simulink model "modules_intentions"  (R2017a)
settings: Solver=ode4  StartTime=0.0  StopTime=time_stop  FixedStep=time_step  RelTol=1e-3
undefined symbols (not defined in the file or in its folder): beta, Delta_guidance, Delta_matrix, eta_initial, initial_desired_psi_vector, initial_desired_u_vector, initial_next_waypoint_indexes, initial_obstacle_ship_states, initial_obstacle_ship_states_dot, initial_reference_psi_vector, initial_reference_u_vector, initial_SBMPC_desired_psi_vector, initial_SBMPC_desired_u_vector, initial_SBMPC_next_waypoint_indexes, initial_SBMPC_obstacle_ship_states, initial_SBMPC_obstacle_ship_states_dot, initial_SBMPC_reference_psi_vector, initial_SBMPC_reference_u_vector, initial_SBMPC_x_d_psi_matrix, initial_SBMPC_x_d_u_matrix, initial_state, initial_x_d_psi_matrix, initial_x_d_u_matrix, K_sway, K_yaw, Kp_feedback_linearization, kp_heading, Nmax, nu_initial, num_obs_ship_waypoints, num_prediction_time_steps, number_of_control_behaviors, number_of_obstacle_ships, number_of_SBMPC_obstacle_ships, obs_speed_between_waypoints, obstacle_waypoint_matrix, Omega_matrix, own_ship_reference_psi_init, own_ship_reference_speed, psi, Psi_init, radius_of_acceptance, SBMPC_obs_speed_between_waypoints, SBMPC_obstacle_waypoint_matrix, seconds_between_prediction, state_vector_init, T, T_k_surge, T_k_sway, T_k_yaw, T_s, T_waypoints, time_step, tsamp, U, U_init, V_init, waypoints_obstacle_ships, waypoints_own_ship, Xmax ... (+1)
(part 4 of 6)

== matlab function modules_intentions/SBMPC obstacle ships/SBMPC using intentions /Calculate control behaviors/Compute hazard ==
  settings: updateMethod=DISCRETE  sampleTime=time_step
  data: obstacle_ships_u_input input size=[1 + number_of_obstacle_ships, num_prediction_time_steps]; obstacle_ships_v_input input size=[1 + number_of_obstacle_ships, num_prediction_time_steps]; obstacle_ships_psi_input input size=[1 + number_of_obstacle_ships, num_prediction_time_steps]; t_0 input; SBMPC_obstacles_own_ship_x_predicted input size=[number_of_SBMPC_obstacle_ships, num_prediction_time_steps, number_of_control_behaviors]; SBMPC_obstacles_own_ship_y_predicted input size=[number_of_SBMPC_obstacle_ships, num_prediction_time_steps, number_of_control_behaviors]; SBMPC_obstacles_own_ship_u_predicted input size=[number_of_SBMPC_obstacle_ships, num_prediction_time_steps, number_of_control_behaviors]; SBMPC_obstacles_own_ship_v_predicted input size=[number_of_SBMPC_obstacle_ships, num_prediction_time_steps, number_of_control_behaviors]; SBMPC_obstacles_own_ship_heading_predicted input size=[number_of_SBMPC_obstacle_ships, num_prediction_time_steps, number_of_control_behaviors]; CLOSE output size=[number_of_SBMPC_obstacle_ships, number_of_control_behaviors, total_number_of_obstacle_ships, num_prediction_time_steps]; d_0 output size=[number_of_SBMPC_obstacle_ships, number_of_control_behaviors, total_number_of_obstacle_ships, num_prediction_time_steps]; obstacle_ships_x_predicted_input input size=[1 + number_of_obstacle_ships, num_prediction_time_steps]; obstacle_ships_y_predicted_input input size=[1 + number_of_obstacle_ships, num_prediction_time_steps]; OVERTAKEN output size=[number_of_SBMPC_obstacle_ships, number_of_control_behaviors, total_number_of_obstacle_ships, num_prediction_time_steps]; STARBOARD output size=[number_of_SBMPC_obstacle_ships, number_of_control_behaviors, total_number_of_obstacle_ships, num_prediction_time_steps]; chosen_HEAD_ON_out output; CROSSED output size=[number_of_SBMPC_obstacle_ships, number_of_control_behaviors, total_number_of_obstacle_ships, num_prediction_time_steps]; mu output size=[number_of_SBMPC_obstacle_ships, number_of_control_behaviors, total_number_of_obstacle_ships, num_prediction_time_steps]; num_prediction_time_steps parameter; heading_angle_offset_commands parameter; propulsion_commands parameter; total_number_of_obstacle_ships parameter; seconds_between_prediction parameter; d_cl parameter; phi_head_on parameter; phi_crossed parameter; phi_overtaken parameter; phi_ahead parameter; K_coll parameter; C output size=[number_of_SBMPC_obstacle_ships, number_of_control_behaviors, total_number_of_obstacle_ships, num_prediction_time_steps]; R output size=[number_of_SBMPC_obstacle_ships, number_of_control_behaviors, total_number_of_obstacle_ships, num_prediction_time_steps]; q parameter; p parameter; d_safe parameter; k_boundary parameter; k_circle parameter; k_Pr parameter; k_psi_port parameter; k_psi_starboard parameter; Delta_Pr parameter; vessel_length parameter; circle_obstacle_parameters parameter; boundary_obstacles_parameters parameter; k_Delta_psi_port parameter; k_Delta_psi_starboard parameter; kappa parameter; f output size=[number_of_SBMPC_obstacle_ships,number_of_control_behaviors]; g output size=[number_of_SBMPC_obstacle_ships,number_of_control_behaviors]; hazard output size=[number_of_SBMPC_obstacle_ships,number_of_control_behaviors]; rad2deg parameter; num_boundary_obstacles parameter; num_circle_obstacles parameter; chosen_C_out output; chosen_P_out output; chosen_FC_out output; chosen_R_out output; chosen_scaled_mu_out output; T_s parameter; chosen_Pr_out output; chosen_psi_ca_out output; C_worst output; R_worst output; scaled_mu_worst output; Pr_worst output; psi_ca_worst output; f_worst_out output; g_worst_out output; smallest_hazard_out output; largest_hazard_out output; f_out output; g_out output; r parameter; L_C input; circle_safety_margin parameter; p_boundary parameter; p_circle parameter; q_circle parameter; q_boundary parameter; boundary_margin parameter; k_role parameter; L_role parameter; ROLE_relative_to_SBMPC_obs_module parameter; L_FC parameter; k_FC parameter; number_of_control_behaviors parameter; HEAD_ON_relative_to_SBMPC_obs_module parameter; chosen_scenario_index_out output; number_of_SBMPC_obstacle_ships parameter; chosen_scenario_index_out_init parameter; data_out_init parameter; number_of_obstacle_ships parameter; HEAD_ON_SBMPC_relative_to_SBMPC_obs parameter; ROLE_SBMPC_relative_to_SBMPC_obs parameter
function [CLOSE, d_0, OVERTAKEN, STARBOARD, chosen_HEAD_ON_out, CROSSED,mu, C, R, f, g, hazard, chosen_C_out, chosen_P_out, chosen_FC_out, chosen_R_out, chosen_scaled_mu_out, chosen_Pr_out, chosen_psi_ca_out, C_worst, R_worst, scaled_mu_worst, Pr_worst, psi_ca_worst, f_worst_out, g_worst_out, smallest_hazard_out, largest_hazard_out, f_out, g_out, chosen_scenario_index_out]                         = computeTotalHazard(obstacle_ships_u_input, obstacle_ships_v_input, obstacle_ships_psi_input, t_0,SBMPC_obstacles_own_ship_x_predicted, SBMPC_obstacles_own_ship_y_predicted,SBMPC_obstacles_own_ship_u_predicted,SBMPC_obstacles_own_ship_v_predicted, SBMPC_obstacles_own_ship_heading_predicted, obstacle_ships_x_predicted_input, obstacle_ships_y_predicted_input, num_prediction_time_steps, heading_angle_offset_commands, propulsion_commands, total_number_of_obstacle_ships, seconds_between_prediction, d_cl,phi_head_on, phi_crossed, phi_overtaken,phi_ahead,K_coll, q, p, d_safe,k_boundary, k_circle, k_Pr, k_psi_port, k_psi_starboard, Delta_Pr, vessel_length, circle_obstacle_parameters, boundary_obstacles_parameters, k_Delta_psi_port, k_Delta_psi_starboard,kappa, rad2deg, num_boundary_obstacles, num_circle_obstacles, T_s, r, L_C,  circle_safety_margin, p_boundary, p_circle, q_circle, q_boundary, boundary_margin, k_role, L_role, ROLE_relative_to_SBMPC_obs_module, L_FC, k_FC, number_of_control_behaviors, HEAD_ON_relative_to_SBMPC_obs_module, number_of_SBMPC_obstacle_ships, chosen_scenario_index_out_init, data_out_init, number_of_obstacle_ships, HEAD_ON_SBMPC_relative_to_SBMPC_obs, ROLE_SBMPC_relative_to_SBMPC_obs)     
    
    persistent chosen_C;
    persistent chosen_scenario_index;
    persistent chosen_R;
    persistent chosen_scaled_mu;
    persistent chosen_P_role;
    persistent chosen_FC;
    persistent chosen_HEAD_ON;
    persistent chosen_Pr;
    persistent chosen_psi_ca;
    persistent chosen_Pr_worst;
    persistent chosen_psi_ca_worst;
    persistent f_worst;
    persistent g_worst;
    persistent f_chosen;
    persistent g_chosen;
    persistent smallest_hazard;
    persistent largest_hazard;
    persistent scenario_index_with_min_hazard;
    persistent scenario_index_with_max_hazard;
    
    if (isempty(chosen_C))
        chosen_C              = zeros(number_of_SBMPC_obstacle_ships,number_of_control_behaviors);%chosen_C_init;
        chosen_scenario_index = ones(1,number_of_SBMPC_obstacle_ships)*7;
        chosen_R              = zeros(number_of_SBMPC_obstacle_ships,number_of_control_behaviors);%chosen_R_init;
        chosen_scaled_mu      = zeros(number_of_SBMPC_obstacle_ships,number_of_control_behaviors);%chosen_scaled_mu_init; 
        chosen_P_role         = zeros(number_of_SBMPC_obstacle_ships,number_of_control_behaviors);%chosen_P_role_init;
        chosen_FC             = zeros(number_of_SBMPC_obstacle_ships,number_of_control_behaviors);
        chosen_HEAD_ON        = zeros(number_of_SBMPC_obstacle_ships,number_of_control_behaviors);
        chosen_Pr             = ones(1, number_of_SBMPC_obstacle_ships);
        chosen_psi_ca         = data_out_init;
        chosen_Pr_worst       = data_out_init;
        chosen_psi_ca_worst   = data_out_init;
        f_worst               = data_out_init;
        g_worst               = data_out_init;
        f_chosen              = data_out_init;
        g_chosen              = data_out_init;
        smallest_hazard       = data_out_init;
        largest_hazard        = data_out_init;
        scenario_index_with_min_hazard = ones(1, number_of_SBMPC_obstacle_ships)*(-1);
        scenario_index_with_max_hazard = ones(1, number_of_SBMPC_obstacle_ships)*(-1);
        
    end
    
    chosen_scenario_index_out = chosen_scenario_index_out_init;

    CLOSE     = zeros(number_of_SBMPC_obstacle_ships, number_of_control_behaviors, total_number_of_obstacle_ships, num_prediction_time_steps);
    OVERTAKEN = zeros(number_of_SBMPC_obstacle_ships, number_of_control_behaviors, total_number_of_obstacle_ships, num_prediction_time_steps);
    STARBOARD = zeros(number_of_SBMPC_obstacle_ships, number_of_control_behaviors, total_number_of_obstacle_ships, num_prediction_time_steps);
    HEAD_ON   = zeros(number_of_SBMPC_obstacle_ships, number_of_control_behaviors, total_number_of_obstacle_ships, num_prediction_time_steps);
    CROSSED   = zeros(number_of_SBMPC_obstacle_ships, number_of_control_behaviors, total_number_of_obstacle_ships, num_prediction_time_steps);
    mu        = zeros(number_of_SBMPC_obstacle_ships, number_of_control_behaviors, total_number_of_obstacle_ships, num_prediction_time_steps);
    scaled_mu = zeros(number_of_SBMPC_obstacle_ships, number_of_control_behaviors, total_number_of_obstacle_ships, num_prediction_time_steps);
    d_0       = zeros(number_of_SBMPC_obstacle_ships, number_of_control_behaviors, total_number_of_obstacle_ships, num_prediction_time_steps);
    f         = zeros(number_of_SBMPC_obstacle_ships,number_of_control_behaviors);
    g         = zeros(number_of_SBMPC_obstacle_ships,number_of_control_behaviors);
    chosen_HEAD_ON_out   = data_out_init;
    chosen_C_out         = data_out_init;
    chosen_P_out         = data_out_init;
    chosen_FC_out        = data_out_init;
    chosen_R_out         = data_out_init;
    chosen_scaled_mu_out =data_out_init;
    chosen_Pr_out        = data_out_init;
    chosen_psi_ca_out    = data_out_init;
    C_worst              = data_out_init;
    P_worst              = data_out_init;
    R_worst              = data_out_init;
    scaled_mu_worst      = data_out_init;
    Pr_worst             = data_out_init;
    psi_ca_worst         =data_out_init;
    f_worst_out          = data_out_init;
    g_worst_out          = data_out_init;
    smallest_hazard_out  = data_out_init;
    largest_hazard_out   = data_out_init;
    f_out                = data_out_init;
    g_out                = data_out_init;
    %R_vector_out         = zeros(number_of_control_behaviors, total_number_of_obstacle_ships, num_prediction_time_steps, number_of_SBMPC_obstacle_ships);
    %chosen_scenario_index_out  = zeros(1, number_of_SBMPC_obstacle_ships);
    %own_ship_u_predicted       = zeros(number_of_SBMPC_obstacle_ships, num_prediction_time_steps, number_of_control_behaviors);
    %own_ship_v_predicted       = zeros(num_prediction_time_steps, number_of_control_behaviors, number_of_SBMPC_obstacle_ships);
    %own_ship_heading_predicted = zeros(num_prediction_time_steps, number_of_control_behaviors, number_of_SBMPC_obstacle_ships);
    %own_ship_x_predicted       = zeros(num_prediction_time_steps, number_of_control_behaviors, number_of_SBMPC_obstacle_ships);
    %own_ship_y_predicted       = zeros(num_prediction_time_steps, number_of_control_behaviors, number_of_SBMPC_obstacle_ships);  
    
    obstacle_ships_u           = zeros(num_prediction_time_steps, total_number_of_obstacle_ships );
    obstacle_ships_v           = zeros(num_prediction_time_steps, total_number_of_obstacle_ships );
    obstacle_ships_psi         = zeros(num_prediction_time_steps, total_number_of_obstacle_ships );
    obstacle_ships_x_predicted = zeros(num_prediction_time_steps, total_number_of_obstacle_ships);
    obstacle_ships_y_predicted = zeros(num_prediction_time_steps, total_number_of_obstacle_ships);
    
    if (num_circle_obstacles > 0)
        g_circle_init  = zeros(number_of_control_behaviors, num_circle_obstacles, num_prediction_time_steps);
    else
        g_circle_init = 0;
    end    
    if (num_boundary_obstacles > 0)
        g_boundary_init = zeros(number_of_control_behaviors, num_boundary_obstacles, num_prediction_time_steps);
    else
        g_boundary_init = 0;
    end 
    g_circle  = g_circle_init;       %3D matrix. 1. dim = scneario, 2. dim = circle obstacle index, 3. dim = prediction horizon time step.
    g_boundary = g_boundary_init;    %3D matrix. 1. dim = scneario, 2. dim = circle obstacle index, 3. dim = prediction horizon time step.
    C = zeros(number_of_SBMPC_obstacle_ships, number_of_control_behaviors, total_number_of_obstacle_ships, num_prediction_time_steps);%C_init; %cost of collision. 3D matrix, 1. dim: scenario, 2. dim: obstacle, 3. dim: prediction horizon time step.
    R = zeros(number_of_SBMPC_obstacle_ships, number_of_control_behaviors, total_number_of_obstacle_ships, num_prediction_time_steps);%R_init; %Risk of collision. 3D matrix, 1. dim: scenario, 2. dim: obstacle, 3. dim: prediction horizon time step.
    hazard = zeros(number_of_SBMPC_obstacle_ships,number_of_control_behaviors); %hazard_init;
    P_role = zeros(number_of_SBMPC_obstacle_ships, number_of_control_behaviors, total_number_of_obstacle_ships, num_prediction_time_steps);%P_role_init;
    FC     = zeros(number_of_SBMPC_obstacle_ships, number_of_control_behaviors, total_number_of_obstacle_ships, num_prediction_time_steps);%FC_init;   
    
    Pr_last = chosen_Pr;     %the Pr corresponding to the previously calculated lowest hazard.
    psi_ca_last = chosen_psi_ca;    
    if (t_0 == 0)
        Pr_last = ones(1, number_of_SBMPC_obstacle_ships);
        psi_ca_last = zeros(1, number_of_SBMPC_obstacle_ships);
    end
    prev_chosen_scenario_index = chosen_scenario_index;
    
    
    ROLE_total    = zeros(number_of_SBMPC_obstacle_ships, total_number_of_obstacle_ships);
    HEAD_ON_total = zeros(number_of_SBMPC_obstacle_ships, total_number_of_obstacle_ships);
    
    if (mod(t_0, seconds_between_prediction) == 0) %only compute every 10th second.
        
        for SBMPC_own_ship_index = 1:number_of_SBMPC_obstacle_ships
           %add SBMPC obstacle ships' data to obsatcle ship data for all sbmpc obstacle vessels except for SBMPC_own_ship_index.
           %obs data: x_predicted, y_predicted, psi, u, v, 
           %obs ship data from function "combine normal obs and own-ship obs ship data" contains own-ship module's vessel data as first element, then normal obs data, and sbmpc obstacle's data can be added at the end. 
           
           index_list = [1:number_of_SBMPC_obstacle_ships];
           SBMPC_obstacle_indexes = index_list(:,[1:(SBMPC_own_ship_index-1),(SBMPC_own_ship_index+1):end]);  %list of index values of all SBMPC obstacles EXCEPT for the SBMPC obstacle chosen to be the own-ship. 
           
           predicted_data_size = size(obstacle_ships_x_predicted_input);
           SBMPC_obs_starting_index = predicted_data_size(1);       % = 1 (own ship) + number of normal obs ships.    
           
           obstacle_ships_u(:,1:SBMPC_obs_starting_index) = obstacle_ships_u_input';
           obstacle_ships_v(:,1:SBMPC_obs_starting_index) = obstacle_ships_v_input';
           obstacle_ships_psi(:,1:SBMPC_obs_starting_index) =obstacle_ships_psi_input';
           obstacle_ships_x_predicted(:,1:SBMPC_obs_starting_index) = obstacle_ships_x_predicted_input';
           obstacle_ships_y_predicted(:,1:SBMPC_obs_starting_index) = obstacle_ships_y_predicted_input';
           
           ROLE_total(SBMPC_own_ship_index, 1:(1+number_of_obstacle_ships))    = ROLE_relative_to_SBMPC_obs_module(:,SBMPC_own_ship_index)';
           HEAD_ON_total(SBMPC_own_ship_index, 1:(1+number_of_obstacle_ships)) = HEAD_ON_relative_to_SBMPC_obs_module(:,SBMPC_own_ship_index)';
          
           if (number_of_SBMPC_obstacle_ships > 1)
               counter = 0;
               for index = 1:length(SBMPC_obstacle_indexes)
                   counter = counter + 1;
                   i = SBMPC_obstacle_indexes(index);
                   obstacle_ships_u(:,SBMPC_obs_starting_index + counter)   = SBMPC_obstacles_own_ship_u_predicted(i,:,prev_chosen_scenario_index(i));
                   obstacle_ships_v(:,SBMPC_obs_starting_index + counter)   = SBMPC_obstacles_own_ship_v_predicted(i,:,prev_chosen_scenario_index(i));
                   obstacle_ships_psi(:,SBMPC_obs_starting_index + counter) = SBMPC_obstacles_own_ship_heading_predicted(i,:,prev_chosen_scenario_index(i));
                   obstacle_ships_x_predicted(:, SBMPC_obs_starting_index + counter) =  SBMPC_obstacles_own_ship_x_predicted(i,:,prev_chosen_scenario_index(i)); %one row for each prediction time step and one column for each ship
                   obstacle_ships_y_predicted(:, SBMPC_obs_starting_index + counter) =  SBMPC_obstacles_own_ship_y_predicted(i,:,prev_chosen_scenario_index(i));   
                   ROLE_total(SBMPC_own_ship_index, 1 + number_of_obstacle_ships + counter)    = ROLE_SBMPC_relative_to_SBMPC_obs(i , SBMPC_own_ship_index);   
                   HEAD_ON_total(SBMPC_own_ship_index, 1 + number_of_obstacle_ships + counter) = HEAD_ON_SBMPC_relative_to_SBMPC_obs(i , SBMPC_own_ship_index);   
               end % end for   
           end
           
           min_ROLE_values = min(ROLE_total(SBMPC_own_ship_index,:));
           %assert (min_ROLE_values(1) >= 0);
           
           own_ship_u_predicted = reshape( SBMPC_obstacles_own_ship_u_predicted(SBMPC_own_ship_index,:,:) , [num_prediction_time_steps, number_of_control_behaviors]);
           own_ship_v_predicted = reshape( SBMPC_obstacles_own_ship_v_predicted(SBMPC_own_ship_index,:,:) , [num_prediction_time_steps, number_of_control_behaviors]);
           own_ship_heading_predicted = reshape( SBMPC_obstacles_own_ship_heading_predicted(SBMPC_own_ship_index,:,:) , [num_prediction_time_steps, number_of_control_behaviors]);
           own_ship_x_predicted = reshape( SBMPC_obstacles_own_ship_x_predicted(SBMPC_own_ship_index,:,:) , [num_prediction_time_steps, number_of_control_behaviors]);
           own_ship_y_predicted = reshape( SBMPC_obstacles_own_ship_y_predicted(SBMPC_own_ship_index,:,:) , [num_prediction_time_steps, number_of_control_behaviors]);
                   
           
           scenario_index = 0;
           for Pr = propulsion_commands
               for psi_ca = heading_angle_offset_commands 
                   scenario_index = scenario_index + 1;                      
                   prediction_time = 0;
                   for t=1:num_prediction_time_steps   
                        prediction_time = t_0 + t*T_s;  
                        %Penalty for static obstacles   
                        if (num_circle_obstacles > 0)
                            circle_obs_counter = 0;
                            for circle_obstacle = circle_obstacle_parameters.'         %in each iteration, circle_obstacle is column vector with [radius; center_x; center_y]
                                circle_obs_counter = circle_obs_counter + 1;
                                radius    = circle_obstacle(1);
                                center_x  = circle_obstacle(2);
                                center_y  = circle_obstacle(3);
                                crossing_with_circle = SBMPC_isCollisionWithCircleObstacle(own_ship_x_predicted(t,scenario_index), own_ship_y_predicted(t,scenario_index), vessel_length, own_ship_heading_predicted(t,scenario_index), center_x, center_y, radius, circle_safety_margin);                       
                                vessel_bow_x = own_ship_x_predicted(t,scenario_index) + cos(own_ship_heading_predicted(t,scenario_index))*(vessel_length/2);
                                vessel_bow_y = own_ship_y_predicted(t,scenario_index) + sin(own_ship_heading_predicted(t,scenario_index))*(vessel_length/2);
                                distance_bow_to_circle_center = sqrt( (center_x - vessel_bow_x)^2 + (center_y - vessel_bow_y)^2 );
                                g_circle(scenario_index, circle_obs_counter, t) = (crossing_with_circle+1)*k_circle*(1/(prediction_time - t_0)^p_circle)*((radius+L_C)/ distance_bow_to_circle_center)^q_circle;%*(psi_ca*rad2deg)     * (1/distance_bow_to_circle_center)                   
                           end % end for circle obs
                        end % end if                        

                        if (num_boundary_obstacles > 0)
                            boundary_obs_counter = 0;
                            for boundary_obstacle = boundary_obstacles_parameters.'
                                boundary_obs_counter = boundary_obs_counter + 1;
                                boundary_start_x = boundary_obstacle(1);
                                boundary_start_y = boundary_obstacle(2);
                                boundary_end_x   = boundary_obstacle(3);
                                boundary_end_y   = boundary_obstacle(4);  
                                vessel_bow_x = own_ship_x_predicted(t,scenario_index) + cos(own_ship_heading_predicted(t,scenario_index))*(vessel_length/2);
                                vessel_bow_y = own_ship_y_predicted(t,scenario_index) + sin(own_ship_heading_predicted(t,scenario_index))*(vessel_length/2);
                                distance_bow_to_line = dist_from_bow_to_line( vessel_bow_x, vessel_bow_y, boundary_start_x, boundary_start_y, boundary_end_x, boundary_end_y ); % from http://paulbourke.net/geometry/pointlineplane/
                                crossing_with_boundary = SBMPC_isCollisionWithBoundaryObstacle(own_ship_x_predicted(t,scenario_index), own_ship_y_predicted(t,scenario_index), vessel_length, own_ship_heading_predicted(t,scenario_index), boundary_start_x, boundary_start_y, boundary_end_x, boundary_end_y);
                                g_boundary(scenario_index, boundary_obs_counter, t) = (crossing_with_boundary+1)*k_boundary*( 1 / (prediction_time - t_0)^p_boundary )*((boundary_margin)/(distance_bow_to_line))^q_boundary;  %from wiki https://en.wikipedia.org/wiki/Distance_from_a_point_to_a_line
                            end % end for boundary obs
                        end % end if
                        
                        for obstacle_ship_index = 1:total_number_of_obstacle_ships
                            obstacle_ship_speed = sqrt(obstacle_ships_u(t,obstacle_ship_index)^2 + obstacle_ships_v(t,obstacle_ship_index)^2);
                            own_ship_speed = sqrt(own_ship_u_predicted(t,scenario_index)^2 + own_ship_v_predicted(t,scenario_index)^2);
                            own_ship_u_NED = own_ship_speed*cos(own_ship_heading_predicted(t,scenario_index));
                            own_ship_v_NED = own_ship_speed*sin(own_ship_heading_predicted(t,scenario_index));
                            obstacle_ship_u_NED = obstacle_ship_speed*cos(obstacle_ships_psi(t,obstacle_ship_index));  
                            obstacle_ship_v_NED = obstacle_ship_speed*sin(obstacle_ships_psi(t,obstacle_ship_index));               
                            V_0 = [own_ship_u_NED,own_ship_v_NED];
                            V_i = [obstacle_ship_u_NED, obstacle_ship_v_NED];       

                            d_0(SBMPC_own_ship_index, scenario_index, obstacle_ship_index, t) = sqrt((own_ship_x_predicted(t,scenario_index) - obstacle_ships_x_predicted(t,obstacle_ship_index))^2 ...
                                                                            +  (own_ship_y_predicted(t,scenario_index) - obstacle_ships_y_predicted(t,obstacle_ship_index))^2); 


                            %%%% CLOSE

                            if (d_0(SBMPC_own_ship_index, scenario_index, obstacle_ship_index, t) <= d_cl(obstacle_ship_index))
                                CLOSE(SBMPC_own_ship_index, scenario_index, obstacle_ship_index, t) = 1;
                            else
                                CLOSE(SBMPC_own_ship_index, scenario_index, obstacle_ship_index, t) = 0;
                            end % end if

                            %%%% OVERTAKEN                  
                            %equation 5 in johansen
                            epsilon = 1;
                            if (CLOSE(SBMPC_own_ship_index, scenario_index, obstacle_ship_index, t) == 1 && obstacle_ship_speed > own_ship_speed + epsilon && dot(V_0, V_i) > cos(phi_overtaken)*norm(V_0)*norm(V_i))
                                OVERTAKEN(SBMPC_own_ship_index, scenario_index, obstacle_ship_index, t) = 1;
                            else
                                OVERTAKEN(SBMPC_own_ship_index, scenario_index, obstacle_ship_index, t) = 0;
                            end % end if

                            %%%% STARBOARD
                            L = [ obstacle_ships_x_predicted(t,obstacle_ship_index) - own_ship_x_predicted(t,scenario_index) , obstacle_ships_y_predicted(t,obstacle_ship_index) - own_ship_y_predicted(t,scenario_index) ];
                            L_unit_vector = L/norm(L);
                            L_angle = atan2(  (obstacle_ships_y_predicted(t,obstacle_ship_index) - own_ship_y_predicted(t,scenario_index)) , (obstacle_ships_x_predicted(t,obstacle_ship_index) - own_ship_x_predicted(t,scenario_index))  );

                            if (L_angle > own_ship_heading_predicted(t,scenario_index))
                                STARBOARD(SBMPC_own_ship_index, scenario_index, obstacle_ship_index, t) = 1;
                            else
                                STARBOARD(SBMPC_own_ship_index, scenario_index, obstacle_ship_index, t) = 0;
                            end
                            %rad2deg = 180/pi;
                            %L_angle_deg = L_angle*rad2deg;
                            %L_angle_deg_converted_to_positive =  mod((L_angle_deg + 360), 360);
                            %L_angle_mapped = L_angle_deg_converted_to_positive*deg2rad;  %map negative angles to positive angles.

                            %%%% HEAD_ON
                            head_on_condition = false;
                            if ( dot(V_0, V_i) < -cos(phi_head_on)*norm(V_0)*norm(V_i) && dot(V_0, L_unit_vector) > cos(phi_ahead)*norm(V_0) ) 
                                head_on_condition = true ; %equation 6-7 in johansen paper 
                            end% end if

                            if (CLOSE(SBMPC_own_ship_index, scenario_index, obstacle_ship_index, t) == 1 && norm(V_i) ~= 0 && head_on_condition == true )
                                HEAD_ON(SBMPC_own_ship_index, scenario_index, obstacle_ship_index, t) = 1;
                            else
                                HEAD_ON(SBMPC_own_ship_index, scenario_index, obstacle_ship_index, t) = 0;
                            end % end if

                            %%%% CROSSED                                              
                            if (CLOSE(SBMPC_own_ship_index, scenario_index, obstacle_ship_index, t) == 1 && dot(V_0, V_i) < cos(phi_crossed)*norm(V_0)*norm(V_i))
                                CROSSED(SBMPC_own_ship_index, scenario_index, obstacle_ship_index, t) = 1;
                            else
                                CROSSED(SBMPC_own_ship_index, scenario_index, obstacle_ship_index, t) = 0;
                            end % end if

                            %%%% RULE14    
                            if (CLOSE(SBMPC_own_ship_index, scenario_index, obstacle_ship_index, t) == 1 && STARBOARD(SBMPC_own_ship_index, scenario_index, obstacle_ship_index, t) == 1 && HEAD_ON(SBMPC_own_ship_index, scenario_index, obstacle_ship_index, t) == 1 )
                                RULE14 = true;
                            else
                                RULE14 = false;
                            end % end if

                            %%%% RULE15   
                            if (CLOSE(SBMPC_own_ship_index, scenario_index, obstacle_ship_index, t) == 1 && STARBOARD(SBMPC_own_ship_index, scenario_index, obstacle_ship_index, t) == 1 && CROSSED(SBMPC_own_ship_index, scenario_index, obstacle_ship_index, t) == 1 && OVERTAKEN(SBMPC_own_ship_index, scenario_index, obstacle_ship_index, t) == 0 )
                                RULE15 = true;
                            else
                                 RULE15 = false;
                            end % end if

                            %%%% mu
                            if (RULE14 || RULE15)
                                mu(SBMPC_own_ship_index, scenario_index, obstacle_ship_index, t) = 1;
                            else
                                mu(SBMPC_own_ship_index, scenario_index, obstacle_ship_index, t) = 0;
                            end % end if                         
                            scaled_mu(SBMPC_own_ship_index, scenario_index, obstacle_ship_index, t) = kappa(obstacle_ship_index)*mu(SBMPC_own_ship_index, scenario_index, obstacle_ship_index, t);


                            %%%% Role variable 
                            if (CLOSE(SBMPC_own_ship_index, scenario_index, obstacle_ship_index, t) == 1 && d_0(SBMPC_own_ship_index, scenario_index, obstacle_ship_index, t) >= L_role)
                                HEAD_ON_intention_value = HEAD_ON_total(SBMPC_own_ship_index,obstacle_ship_index);
                                P_role(SBMPC_own_ship_index, scenario_index, obstacle_ship_index, t) = ROLE_total(SBMPC_own_ship_index,obstacle_ship_index)*k_role*(1-HEAD_ON_intention_value)*(sqrt(abs(psi_ca*rad2deg)) + 1 - Pr);        
                            else
                                P_role(SBMPC_own_ship_index, scenario_index, obstacle_ship_index, t) = 0;
                            end % end if



                            %%%% Cost of collision
                            C(SBMPC_own_ship_index, scenario_index, obstacle_ship_index, t) = K_coll(obstacle_ship_index)*norm(V_0 - V_i)^2;

                            %%%% Risk of collision    

                            if (d_0(SBMPC_own_ship_index, scenario_index, obstacle_ship_index, t) <= L_FC)
                                FC(SBMPC_own_ship_index, scenario_index, obstacle_ship_index, t) = 1;
                            else
                                FC(SBMPC_own_ship_index, scenario_index, obstacle_ship_index, t) = 0;
                            end % end if


                            if (d_0(SBMPC_own_ship_index, scenario_index, obstacle_ship_index, t) <= d_safe(obstacle_ship_index) && d_0(SBMPC_own_ship_index, scenario_index, obstacle_ship_index, t) >= 20)                          
                                R(SBMPC_own_ship_index, scenario_index, obstacle_ship_index, t)  = (1 / (abs(prediction_time - t_0)^p))*( r*( d_safe(obstacle_ship_index) / d_0(SBMPC_own_ship_index, scenario_index, obstacle_ship_index, t) )^q  + k_FC*FC(SBMPC_own_ship_index, scenario_index, obstacle_ship_index, t)   ) ;
                                if ( R(SBMPC_own_ship_index, scenario_index, obstacle_ship_index, t) >= 20000)
                                    R(SBMPC_own_ship_index, scenario_index, obstacle_ship_index, t) = 20000;  %saturate
                                end
                            else
                                R(SBMPC_own_ship_index, scenario_index, obstacle_ship_index, t) = 0;
                            end % end if        

                        end % end for - num obs ships        
                   end % end for t
               end % end for psi_ca
            end % end for Pr
           
            scenario_index = 0;
            for Pr = propulsion_commands
                for psi_ca = heading_angle_offset_commands 
                    scenario_index = scenario_index + 1;
                    sum_matrix = C(SBMPC_own_ship_index,scenario_index,:,:).*R(SBMPC_own_ship_index, scenario_index,:,:) + scaled_mu(SBMPC_own_ship_index, scenario_index,:,:) + P_role(SBMPC_own_ship_index,scenario_index,:,:);   
                    sum_matrix = reshape(sum_matrix, total_number_of_obstacle_ships, num_prediction_time_steps);
                    [best_value,idx] = max(sum_matrix(:));
                    [best_obstacle_ship_index,best_timestep] = ind2sub(size(sum_matrix),idx);                          

                    if ( psi_ca < 0)
                        k_psi = k_psi_port;  
                        Delta_psi = k_Delta_psi_port*(abs(psi_ca*rad2deg - psi_ca_last(SBMPC_own_ship_index)*rad2deg));
                    else
                        k_psi = k_psi_starboard;
                        Delta_psi = k_Delta_psi_starboard*(abs(psi_ca*rad2deg - psi_ca_last(SBMPC_own_ship_index)*rad2deg));
                    end % end if                

                    f(SBMPC_own_ship_index, scenario_index) = k_Pr*(1-Pr) + k_psi*(abs(psi_ca*rad2deg)) + Delta_Pr*abs(Pr - Pr_last(SBMPC_own_ship_index)) + Delta_psi ;                                 

                    g_circle_scenario = 0;
                    if (num_circle_obstacles > 0)
                        g_circle_scenario_values = g_circle(scenario_index, :, :);
                        g_circle_scenario = max(g_circle_scenario_values(:));
                    end % end if                
                    g_boundary_scenario = 0;
                    if (num_boundary_obstacles > 0)
                        g_boundary_scenario_values = g_boundary(scenario_index, :, :);
                        g_boundary_scenario = max(g_boundary_scenario_values(:));
                    end % end if                
                    g(SBMPC_own_ship_index, scenario_index) = g_circle_scenario + g_boundary_scenario;

                    hazard(SBMPC_own_ship_index, scenario_index) = best_value + f(SBMPC_own_ship_index, scenario_index) + g(SBMPC_own_ship_index, scenario_index);

                    %The C, R and K*µ corresponding to the values used to find hazard H for scenario k.
                    chosen_C(SBMPC_own_ship_index, scenario_index) = C(SBMPC_own_ship_index,scenario_index,best_obstacle_ship_index,best_timestep);  %the C value used to compute hazard in scenario number "scenario_index"
                    chosen_R(SBMPC_own_ship_index, scenario_index) = R(SBMPC_own_ship_index,scenario_index,best_obstacle_ship_index,best_timestep);

                    chosen_scaled_mu(SBMPC_own_ship_index, scenario_index) = scaled_mu(SBMPC_own_ship_index, scenario_index,best_obstacle_ship_index,best_timestep);  
                    chosen_P_role(SBMPC_own_ship_index, scenario_index) = P_role(SBMPC_own_ship_index, scenario_index,best_obstacle_ship_index,best_timestep);
                    chosen_FC(SBMPC_own_ship_index, scenario_index)     = FC(SBMPC_own_ship_index, scenario_index,best_obstacle_ship_index,best_timestep)*k_FC;

                    chosen_HEAD_ON(SBMPC_own_ship_index, scenario_index) = HEAD_ON(SBMPC_own_ship_index, scenario_index, best_obstacle_ship_index, best_timestep);

                    assert (best_value == chosen_C(SBMPC_own_ship_index, scenario_index)*chosen_R(SBMPC_own_ship_index, scenario_index) + chosen_scaled_mu(SBMPC_own_ship_index, scenario_index) + chosen_P_role(SBMPC_own_ship_index, scenario_index));                                           
                end % end for
            end % end for
            
            [min_hazard, scenario_index_with_min_hazard] = min(hazard(SBMPC_own_ship_index,:));
            [max_hazard, scenario_index_with_max_hazard] = max(hazard(SBMPC_own_ship_index,:));  
            smallest_hazard(SBMPC_own_ship_index) = min_hazard;
            largest_hazard(SBMPC_own_ship_index) = max_hazard;

            %h_min = hazard(SBMPC_own_ship_index,scenario_index_with_min_hazard);
            %h_max = hazard(SBMPC_own_ship_index,scenario_index_with_max_hazard);
            %assert(min_hazard == hazard(SBMPC_own_ship_index,scenario_index_with_min_hazard));
            %assert(max_hazard == h_max);

            f_chosen(SBMPC_own_ship_index) = f(SBMPC_own_ship_index, scenario_index_with_min_hazard);
            g_chosen(SBMPC_own_ship_index) = g(SBMPC_own_ship_index, scenario_index_with_min_hazard);
            f_worst(SBMPC_own_ship_index)  = f(SBMPC_own_ship_index, scenario_index_with_max_hazard);
            g_worst(SBMPC_own_ship_index)  = g(SBMPC_own_ship_index, scenario_index_with_max_hazard); 

            scenario_index = 0;
            for Pr = propulsion_commands
                for psi_ca = heading_angle_offset_commands
                    scenario_index = scenario_index +1;
                    if (scenario_index == scenario_index_with_min_hazard)
                        chosen_Pr(SBMPC_own_ship_index) = Pr;
                        chosen_psi_ca(SBMPC_own_ship_index) = psi_ca; 
                        chosen_scenario_index(SBMPC_own_ship_index) = scenario_index;
                    elseif (scenario_index == scenario_index_with_max_hazard)
                        chosen_Pr_worst(SBMPC_own_ship_index) = Pr;
                        chosen_psi_ca_worst(SBMPC_own_ship_index) = psi_ca;                   
                    end % end if
                end % end for
            end % end for               
         end % end for sbmpc obstacles                  
     end % end if
    
     
    for i = 1:number_of_SBMPC_obstacle_ships
        chosen_C_out(i) = chosen_C(i);
        chosen_scenario_index_out(i) = chosen_scenario_index(i);
        chosen_P_out(i) = chosen_P_role(i);
        chosen_FC_out(i) = chosen_FC(i);
        chosen_HEAD_ON_out(i) = chosen_HEAD_ON(i);
        C_worst(i) = chosen_C(i);
        P_worst(i) = chosen_P_role(i);
        chosen_R_out(i) = chosen_R(i);
        R_worst(i) = chosen_R(i);
        chosen_scaled_mu_out(i) = chosen_scaled_mu(i);
        scaled_mu_worst(i) = chosen_scaled_mu(i);
        chosen_Pr_out(i) = chosen_Pr(i);
        Pr_worst(i) = chosen_Pr_worst(i);
        chosen_psi_ca_out(i) = chosen_psi_ca(i);
        psi_ca_worst(i) = chosen_psi_ca_worst(i);
        f_worst_out(i) = f_worst(i);
        g_worst_out(i) = g_worst(i);
        %R_vector_out(i) = R(SBMPC_own_ship_index,:, :, :);

        f_out(i) = f_chosen(i);
        g_out(i) = g_chosen(i);
        smallest_hazard_out(i) = smallest_hazard(i);
        largest_hazard_out(i) =  largest_hazard(i);   
    end
    
     
    

 end % end function

== matlab function modules_intentions/Own-ship/SBMPC USING INTENTIONS /Normal obstacle ships trajectories prediction/Normal obstacle ships trajectories prediction ==
  settings: updateMethod=DISCRETE  sampleTime=time_step
  data: obstacle_ships_headings input; obstacle_ships_x_predicted output size=[num_prediction_time_steps, number_of_obstacle_ships]; obstacle_ships_y_predicted output size=[num_prediction_time_steps, number_of_obstacle_ships]; obstacle_ships_next_waypoint_index_vector input; obstacle_ships_initial_positions input; T_s parameter; t_0 input; number_of_obstacle_ships parameter; T parameter; seconds_between_prediction parameter; num_prediction_time_steps parameter; num_obs_ship_waypoints parameter; waypoints_obstacle_ships parameter; U parameter; psi parameter; T_waypoints parameter; obstacle_ships_u_predicted output size=[num_prediction_time_steps, number_of_obstacle_ships]; obstacle_ships_v_predicted output size=[num_prediction_time_steps, number_of_obstacle_ships]; obstacle_ships_psi_predicted output size=[num_prediction_time_steps, number_of_obstacle_ships]
function [obstacle_ships_x_predicted,obstacle_ships_y_predicted, obstacle_ships_u_predicted, obstacle_ships_v_predicted, obstacle_ships_psi_predicted] = normalObstacleShipsTrajectoryPrediction(obstacle_ships_headings, obstacle_ships_next_waypoint_index_vector, obstacle_ships_initial_positions, T_s, t_0, number_of_obstacle_ships, T, seconds_between_prediction, num_prediction_time_steps, num_obs_ship_waypoints, waypoints_obstacle_ships, U, psi, T_waypoints)
     deg2rad = pi/180;
     rad2deg = 180/pi;
     obstacle_ships_x_predicted = zeros( num_prediction_time_steps, number_of_obstacle_ships);   % obstacle_ships_x_predicted_init;  %%each row is a point in time, each column is an obstacle
     obstacle_ships_y_predicted = zeros( num_prediction_time_steps, number_of_obstacle_ships);   %obstacle_ships_y_predicted_init;  %%each row is a point in time, each column is an obstacle    
     obstacle_ships_u_predicted = zeros( num_prediction_time_steps, number_of_obstacle_ships);
     obstacle_ships_v_predicted = zeros( num_prediction_time_steps, number_of_obstacle_ships);
     obstacle_ships_psi_predicted = zeros( num_prediction_time_steps, number_of_obstacle_ships);
     if (mod(t_0, seconds_between_prediction) == 0)                 %Only do calculation every "seconds_between_prediction" second.
         for obstacle_ship_index = 1:number_of_obstacle_ships
             next_wp_index_at_t0 = obstacle_ships_next_waypoint_index_vector(obstacle_ship_index); 
             next_wp_index = next_wp_index_at_t0;
             obs_waypoints = waypoints_obstacle_ships(:,:,obstacle_ship_index); 
             obs_x_init = obstacle_ships_initial_positions(obstacle_ship_index, 1);
             obs_y_init = obstacle_ships_initial_positions(obstacle_ship_index, 2);
             prediction_time =  - T_s; %reset value  
             T_changed_wp = 0;
             obs_x_when_changed_wp = obs_x_init;
             obs_y_when_changed_wp = obs_y_init;
             change_wp_index_bool = true;
             for t = 1:num_prediction_time_steps  
                prediction_time = prediction_time + T_s;
                U_hat   = U(obstacle_ship_index, next_wp_index-1);
                %psi_hat = psi(obstacle_ship_index, next_wp_index-1);
                obstacle_ships_u_predicted(t, obstacle_ship_index) = U_hat;
                obstacle_ships_v_predicted(t, obstacle_ship_index) = 0;
                
                
                if (next_wp_index_at_t0 == num_obs_ship_waypoints)
                    psi_hat = psi(obstacle_ship_index, num_obs_ship_waypoints-1);
                    obstacle_ships_x_predicted(t, obstacle_ship_index) = obs_x_init + U_hat*cos(psi_hat)*prediction_time;
                    obstacle_ships_y_predicted(t, obstacle_ship_index) = obs_y_init + U_hat*sin(psi_hat)*prediction_time;
                    obstacle_ships_psi_predicted(t, obstacle_ship_index) = psi_hat;
                
                elseif (next_wp_index == next_wp_index_at_t0)
                    psi_hat = atan2(obs_waypoints(next_wp_index, 2) - obs_y_when_changed_wp    ,  obs_waypoints(next_wp_index, 1) - obs_x_when_changed_wp );
                    if  (  abs(psi_hat*rad2deg - obstacle_ships_headings(obstacle_ship_index)*rad2deg) >= 30 && next_wp_index >= 3 && change_wp_index_bool)
                        next_wp_index = next_wp_index -1;
                        next_wp_index_at_t0 = next_wp_index_at_t0 - 1;
                        change_wp_index_bool = false;
                        psi_hat = atan2(obs_waypoints(next_wp_index, 2) - obs_y_when_changed_wp    ,  obs_waypoints(next_wp_index, 1) - obs_x_when_changed_wp );
                    end 
                    obstacle_ships_psi_predicted(t, obstacle_ship_index) = psi_hat;
                    obstacle_ships_x_predicted(t, obstacle_ship_index) = obs_x_init + U_hat*cos(psi_hat)*prediction_time;
                    obstacle_ships_y_predicted(t, obstacle_ship_index) = obs_y_init + U_hat*sin(psi_hat)*prediction_time;
                elseif (next_wp_index > next_wp_index_at_t0 && next_wp_index <= num_obs_ship_waypoints) 
                    psi_hat = atan2(obs_waypoints(next_wp_index, 2) - obs_y_when_changed_wp    ,  obs_waypoints(next_wp_index, 1) - obs_x_when_changed_wp );
                    obstacle_ships_psi_predicted(t, obstacle_ship_index) = psi_hat;
                    obstacle_ships_x_predicted(t, obstacle_ship_index) = obs_x_when_changed_wp + U_hat*cos(psi_hat)*(prediction_time - T_changed_wp);
                    obstacle_ships_y_predicted(t, obstacle_ship_index) = obs_y_when_changed_wp + U_hat*sin(psi_hat)*(prediction_time - T_changed_wp);
                end % end if
                if ( obstacle_ships_psi_predicted(t, obstacle_ship_index) == 180*deg2rad)
                    obstacle_ships_psi_predicted(t, obstacle_ship_index) = -180*deg2rad;
                end
                
                dist_to_next_wp = sqrt( (obstacle_ships_x_predicted(t, obstacle_ship_index) - obs_waypoints(next_wp_index, 1) )^2 + ( obstacle_ships_y_predicted(t, obstacle_ship_index) - obs_waypoints(next_wp_index, 2)  )^2 ); 
              
                if (dist_to_next_wp <= 50 && next_wp_index ~= num_obs_ship_waypoints)
                    next_wp_index = next_wp_index + 1;   
                    T_changed_wp = prediction_time;
                    %%%%psi_hat = obstacle_ships_headings(obstacle_ship_index);
                    obs_x_when_changed_wp = obstacle_ships_x_predicted(t, obstacle_ship_index);
                    obs_y_when_changed_wp = obstacle_ships_y_predicted(t, obstacle_ship_index);
                end % end if
                

             end % end for
         end % end for
     end % end if

end

== matlab function modules_intentions/Own-ship/guidance/waypoint guidance ==
  data: waypoints input; reference_psi output; vessel_position input; time_step parameter; beta parameter; Delta_guidance parameter; radius_of_acceptance parameter; next_waypoint_index output; own_ship_reference_psi_init parameter
function [reference_psi,next_waypoint_index]  = waypoint_guidance(waypoints, vessel_position, time_step, beta, Delta_guidance, radius_of_acceptance, own_ship_reference_psi_init)
    persistent waypointGuidanceObject;
    
    if (isempty(waypointGuidanceObject))
        waypointGuidanceObject = waypointGuidance_class(own_ship_reference_psi_init, waypoints, vessel_position, Delta_guidance, beta, time_step, radius_of_acceptance);
    end
    
    waypointGuidanceObject = waypointGuidanceObject.updateVesselPosition(vessel_position);
    waypointGuidanceObject = waypointGuidanceObject.updateCurrentWaypoint();
    [waypointGuidanceObject, reference_psi] = waypointGuidanceObject.getReferencePsi();    
    next_waypoint_index = waypointGuidanceObject.getNextwaypointIndex();
end

== matlab function modules_intentions/Own-ship/reference model nu/MATLAB Function ==
  data: reference_u input; nu_initial parameter; time_step parameter; x_d_new output; Delta_matrix parameter; Omega_matrix parameter
function x_d_new = ReferenceModelForSpeed(reference_u, nu_initial, time_step, Delta_matrix, Omega_matrix)    

persistent x_d %[nu; nu_dot] = [u,v,r, u_dot, v_dot, r_dot]

if isempty(x_d)
    x_d = [nu_initial;0;0;0];
end

x_d = speedReferenceModel(x_d, reference_u, time_step, Delta_matrix, Omega_matrix);
x_d_new = x_d;
end
